simulink model "EjemploServidorConPioneerM2011b"  (Simulink 7.8)
settings: Solver=ode3  StartTime=0.0  StopTime=inf  FixedStep=0.001  RelTol=1e-3
libraries: aerolibanimutils x1
settings Model: Creator=Usuario  LastModifiedBy=Sebastián
settings OptimizationCC: SimCompilerOptimization=On
settings CodeAppCC: CustomSymbolStrType=$N$R$M_T

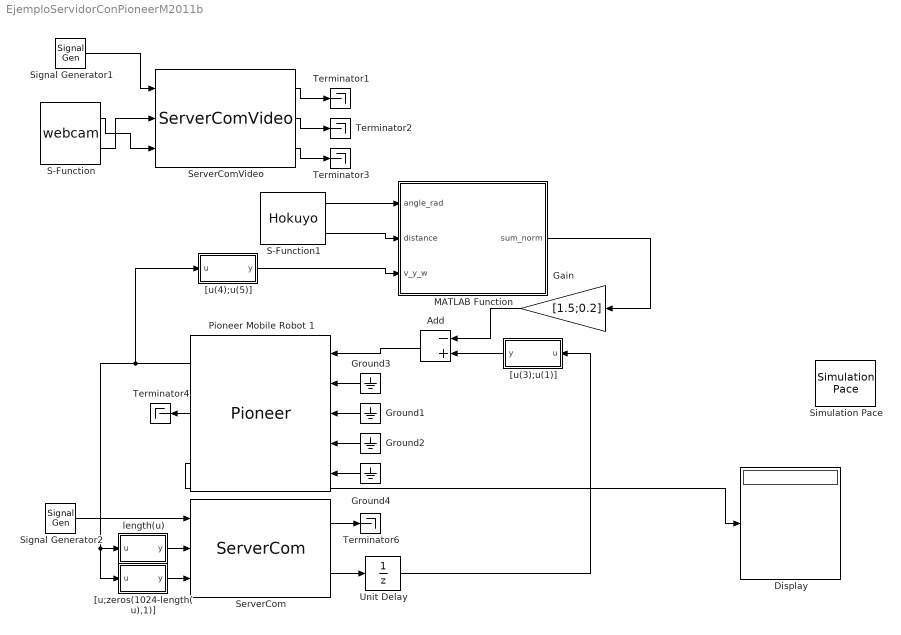
== system EjemploServidorConPioneerM2011b ==
  Add : Sum  Inputs=-+
  Display : Display
  Gain : Gain  Gain=[1.5;0.2]
  Ground{1..4} (4 alike) : Ground
  MATLAB Function : MATLAB Function  TreatAsAtomicUnit=on
  Pioneer Mobile Robot 1 : S-Function  FunctionName=Pioneer  Parameters=1  EnableBusSupport=off
      mask Display:
      | color('red')
      | port_label('input',1,'acciones')
      | port_label('input',2,'postura')
      | port_label('input',3,'parametros')
      | port_label('input',4,'parametrosSend')
      | port_label('input',5,'posturaSend')
      | color('blue')
      | port_label('output',1,'estado')
      | port_label('output',2,'parametros')
      | port_label('output',3,'laser')
  S-Function : S-Function  FunctionName=webcam  Parameters=1  EnableBusSupport=off
  S-Function1 : S-Function  FunctionName=Hokuyo  EnableBusSupport=off
  ServerCom : S-Function  FunctionName=ServerCom  EnableBusSupport=off
      mask Display:
      | patch([0 4. 4 0],[0.02 0.02 0.98 0.98],0.9*[123 193 255]/255)
      | patch([0 4 4 0],[0.1 0.1 0.9 0.9],[123 193 255]/255)
      | patch([1.5 2.5 2.5 2.3 2.3 1.7 1.7 1.5],[0 0 1 1 1.2 1.2 1 1],[130 130 130]/255)
      | patch([1.3 2.7 2.7 1.3],[1.2 1.2 2.9 2.9],0.85*[130 130 130]/255)
      | patch([1.4 2.6 2.6 1.4],[1.3 1.3 2.8 2.8],[123 193 255]/255)
      | patch([1.5 2.5 2.5 1.5],[1.4 1.4 2.7 2.7],0.85*[130 130 130]/255)
      | patch([1.9 2.1 2.1 1.9],[1.8 1.8 2.1 2.1],[123 193 255]/255)
      | color('red')
      | port_label('input',1,'clock')
      | port_label('input',2,'sizeSend')
      | port_label('input',3,'dataSend')
      | port_label('output',1,'stateChannel')
      | port_label('output',2,'dataRecv')
  ServerComVideo : S-Function  FunctionName=ServerComVideo  EnableBusSupport=off
      mask Display:
      | patch([0 4. 4 0],[0.02 0.02 0.98 0.98],0.9*[123 193 255]/255)
      | patch([0 4 4 0],[0.1 0.1 0.9 0.9],[123 193 255]/255)
      | patch([1.5 2.5 2.5 2.3 2.3 1.7 1.7 1.5],[0 0 1 1 1.2 1.2 1 1],[130 130 130]/255)
      | patch([1.3 2.7 2.7 1.3],[1.2 1.2 2.9 2.9],0.85*[130 130 130]/255)
      | patch([1.4 2.6 2.6 1.4],[1.3 1.3 2.8 2.8],[123 193 255]/255)
      | patch([1.5 2.5 2.5 1.5],[1.4 1.4 2.7 2.7],0.85*[130 130 130]/255)
      | patch([1.9 2.1 2.1 1.9],[1.8 1.8 2.1 2.1],[123 193 255]/255)
      | color('red')
      | port_label('input',1,'clock')
      | port_label('input',2,'sizeSend')
      | port_label('input',3,'dataSend')
      | port_label('output',1,'stateChannel')
      | port_label('output',2,'sizeMustBeRecv')
      | port_label('output',3,'dataRecv')
  Signal Generator1 : SignalGenerator  WaveForm=square  Frequency=20
  Signal Generator2 : SignalGenerator  WaveForm=square  Frequency=20
  Simulation Pace : aerolibanimutils/Simulation Pace  SimulationPace=1  SleepMode=MATLAB Thread  OutputPaceError=off  SampleTime=-1
      settings: AttributesFormatString=%<SimulationPace> sec/sec
  Terminator{1..4,6} (5 alike) : Terminator
  Unit Delay : UnitDelay  SampleTime=-1
  "[u(3);u(1)]" : MATLAB Function  TreatAsAtomicUnit=on
  "[u(4);u(5)]" : MATLAB Function  TreatAsAtomicUnit=on
  "[u;zeros(1024-length(u),1)]" : MATLAB Function  TreatAsAtomicUnit=on
  length(u) : MATLAB Function  TreatAsAtomicUnit=on
  wires:
  Signal Generator1/1 -> ServerComVideo/1
  S-Function/2 -> ServerComVideo/2
  S-Function/1 -> ServerComVideo/3
  ServerComVideo/1 -> Terminator1/1
  ServerComVideo/2 -> Terminator2/1
  ServerComVideo/3 -> Terminator3/1
  "[u;zeros(1024-length(u),1)]"/1(y) -> ServerCom/3
  Pioneer Mobile Robot 1/1 -> "[u;zeros(1024-length(u),1)]"/1(u), length(u)/1(u), "[u(4);u(5)]"/1(u)
  Signal Generator2/1 -> ServerCom/1
  length(u)/1(y) -> ServerCom/2
  Pioneer Mobile Robot 1/2 -> Terminator4/1
  Pioneer Mobile Robot 1/3 -> Display/1
  Ground3/1 -> Pioneer Mobile Robot 1/2
  Ground1/1 -> Pioneer Mobile Robot 1/3
  Ground2/1 -> Pioneer Mobile Robot 1/4
  Ground4/1 -> Pioneer Mobile Robot 1/5
  ServerCom/2 -> Unit Delay/1
  ServerCom/1 -> Terminator6/1
  Unit Delay/1 -> "[u(3);u(1)]"/1(u)
  S-Function1/1 -> MATLAB Function/1(angle_rad)
  "[u(4);u(5)]"/1(y) -> MATLAB Function/3(v_y_w)
  S-Function1/3 -> MATLAB Function/2(distance)
  "[u(3);u(1)]"/1(y) -> Add/2
  Add/1 -> Pioneer Mobile Robot 1/1
  MATLAB Function/1(sum_norm) -> Gain/1
  Gain/1 -> Add/1

== matlab function length(u) ==
  data: u input double; y output double
function y = fcn(u)
%#codegen

y = uint32(length(u));

== matlab function [u;zeros(1024-length(u),1)] ==
  data: u input double; y output double
function y = fcn(u)
%#codegen

y = [u;zeros(1024-length(u),1)];

== matlab function [u(3);u(1)] ==
  data: u input double; y output double
function y = fcn(u)
%#codegen

y = [u(3);u(1)];

== matlab function MATLAB Function ==
  data: angle_rad input double; distance input double; sum_norm output double; v_y_w input double
function sum_norm = fcn(angle_rad,distance,v_y_w)
%#codegen

delta=0.3;
c=0.4;
s_max=1.5;
s_min=0.2;

if((abs(v_y_w(2))<0.0001))
    r=10000;
else
    r=abs(v_y_w(1))/abs(v_y_w(2));
end


if(v_y_w(2)>=0)
    xR=r;
else
    xR=-r;
end

xc=zeros(4,1);
yc=zeros(4,1);

sum=0;
p=0;

count=0;

for i=86:598
    
    if(distance(i)<4)
        xl=-distance(i)*sin(angle_rad(i))+xR;
        yl=distance(i)*cos(angle_rad(i));
        
        xc(1)=r*xl/sqrt(xl^2+yl^2);
        xc(2)=-r*xl/sqrt(xl^2+yl^2);
        xc(3)=r*xl/sqrt(xl^2+yl^2);
        xc(4)=-r*xl/sqrt(xl^2+yl^2);
        yc(1)=sqrt(r^2-xc(1)^2);
        yc(2)=sqrt(r^2-xc(2)^2);
        yc(3)=-sqrt(r^2-xc(3)^2);
        yc(4)=-sqrt(r^2-xc(4)^2);

        d=sqrt((xl-xc).^2+(yl-yc).^2);
        [d,j]=min(d);
           
        tita=atan2(yc(j),xc(j));
        if(v_y_w(2)<0) 
            tita=pi-tita;
        end
        
        s=r*tita;
        
        if(s<s_max)
            
            if(d<=(c/2))
                p=1;
                count=count+1;
            end
            if((d>(c/2))&&(d<(delta+c/2)))
                  p=(1+cos((pi/delta)*(d-(c/2))))/2;
                  count=count+1;
            end
            if(d>=(delta+c/2))
                p=0;
            end
            
            if(s<s_min)
                s=s_min;
            end
            
            sum=sum+p*(s_max-s);
            
        end
        
    end
    
end

sum_norm=sum/((s_max-s_min)*513); %513 es la cantidad de lasers de -90 (laser 86) a 90 (laser 598) grado
sum_norm=sqrt(sum_norm);

== matlab function [u(4);u(5)] ==
  data: u input double; y output double
function y = fcn(u)
%#codegen

y = [u(4);u(5)];
